simulink model "Optimate_PhysicalArchi"  (R2022b)
settings: Solver=VariableStepAuto  StartTime=0.0  StopTime=10.0  RelTol=1e-3
settings Model: DataDictionary=Optimate_PhysicalArchiDD.sldd  Creator=TO41629  LastModifiedBy=TO41629

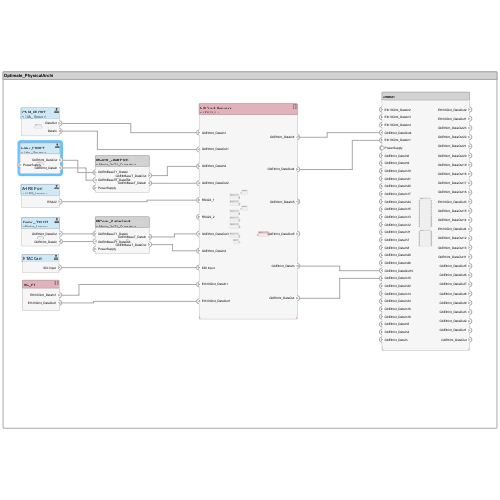
[thumbnail: Simulink's stored preview of the top-level diagram]
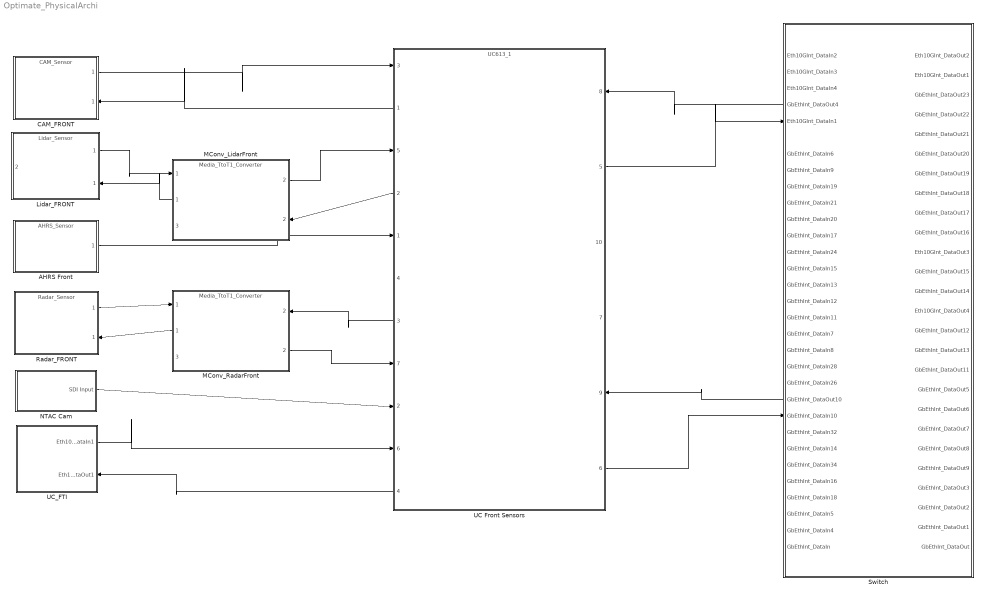
== system Optimate_PhysicalArchi ==
  AHRS Front : ModelReference  ModelNameDialog=AHRS_Sensor  SimulationMode=Normal  ModelReferenceVersion=1.2
      settings: PortSchema="{\"entries\":[{\"content\":{\"headerSize\":38,\"margin\":15,\"minimumSpacing\":25,\"sides\":[{\"content\":{\"connectorIds\":[]},\"type\":\"ConnectorPlacement.EquallySpacedRectSide\",\"uuid\":\"c7a9dcc5-4699-4aa5-9b03-01cd9c9d5d35\"},{\"content\":{\"connectorIds\":[\"Out1\"],\"side\":\"RIGHT\"},\"type\":\"ConnectorPlacement.EquallySpacedRectSide\",\"uuid\":\"7085d3c2-4a9c-4f60-a450-73088e37e883\"},{\"content\":{\"connectorIds\":[],\"side\":\"TOP\"},\"type\":\"ConnectorPlacement.EquallySpacedRectSide\",\"uuid\":\"b1aea649-404c-4f50-816f-0908c9ccfd50\"}]},\"type\":\"ConnectorPlacement.EquallySpacedConnector\",\"uuid\":\"4d292e22-38cf-4a1e-b63b-51fd039b5bd2\"}],\"packageUris\":[\"http://schema.mathworks.com/mf0/Connector/R2020b\"],\"version\":\"1.0\"}"
  CAM_FRONT : ModelReference  ModelNameDialog=CAM_Sensor  UsingDefaultArgumentValue=0,0,0,0,0  SimulationMode=Normal  ModelReferenceVersion=1.17
      settings: PortSchema="{\"entries\":[{\"content\":{\"headerSize\":38,\"margin\":15,\"minimumSpacing\":25,\"sides\":[{\"content\":{\"connectorIds\":[]},\"type\":\"ConnectorPlacement.EquallySpacedRectSide\",\"uuid\":\"c7a9dcc5-4699-4aa5-9b03-01cd9c9d5d35\"},{\"content\":{\"connectorIds\":[\"Out1\",\"In1\"],\"side\":\"RIGHT\"},\"type\":\"ConnectorPlacement.EquallySpacedRectSide\",\"uuid\":\"7085d3c2-4a9c-4f60-a450-73088e37e883\"},{\"content\":{\"connectorIds\":[],\"side\":\"TOP\"},\"type\":\"ConnectorPlacement.EquallySpacedRectSide\",\"uuid\":\"b1aea649-404c-4f50-816f-0908c9ccfd50\"}]},\"type\":\"ConnectorPlacement.EquallySpacedConnector\",\"uuid\":\"4d292e22-38cf-4a1e-b63b-51fd039b5bd2\"}],\"packageUris\":[\"http://schema.mathworks.com/mf0/Connector/R2020b\"],\"version\":\"1.0\"}"
  Lidar_FRONT : ModelReference  ModelNameDialog=Lidar_Sensor  SimulationMode=Normal  ModelReferenceVersion=1.6
      settings: PortSchema="{\"entries\":[{\"content\":{\"headerSize\":38,\"margin\":15,\"minimumSpacing\":25,\"sides\":[{\"content\":{\"connectorIds\":[\"In2\"]},\"type\":\"ConnectorPlacement.EquallySpacedRectSide\",\"uuid\":\"c7a9dcc5-4699-4aa5-9b03-01cd9c9d5d35\"},{\"content\":{\"connectorIds\":[\"Out1\",\"In1\"],\"side\":\"RIGHT\"},\"type\":\"ConnectorPlacement.EquallySpacedRectSide\",\"uuid\":\"7085d3c2-4a9c-4f60-a450-73088e37e883\"},{\"content\":{\"connectorIds\":[],\"side\":\"TOP\"},\"type\":\"ConnectorPlacement.EquallySpacedRectSide\",\"uuid\":\"b1aea649-404c-4f50-816f-0908c9ccfd50\"}]},\"type\":\"ConnectorPlacement.EquallySpacedConnector\",\"uuid\":\"4d292e22-38cf-4a1e-b63b-51fd039b5bd2\"}],\"packageUris\":[\"http://schema.mathworks.com/mf0/Connector/R2020b\"],\"version\":\"1.0\"}"
  MConv_LidarFront : ModelReference  ModelNameDialog=Media_TtoT1_Converter  SimulationMode=Normal  ModelReferenceVersion=1.4
      settings: PortSchema="{\"entries\":[{\"content\":{\"headerSize\":38,\"margin\":15,\"minimumSpacing\":25,\"sides\":[{\"content\":{\"connectorIds\":[\"In1\",\"Out1\",\"In3\"]},\"type\":\"ConnectorPlacement.EquallySpacedRectSide\",\"uuid\":\"99f9264f-b53d-4971-8b33-a510fd21d3a3\"},{\"content\":{\"connectorIds\":[\"Out2\",\"In2\"],\"side\":\"RIGHT\"},\"type\":\"ConnectorPlacement.EquallySpacedRectSide\",\"uuid\":\"2d9ba29c-7f97-48cb-9608-186fea073d48\"},{\"content\":{\"connectorIds\":[],\"side\":\"TOP\"},\"type\":\"ConnectorPlacement.EquallySpacedRectSide\",\"uuid\":\"4aabfdd9-8cc9-4862-a428-8fddf83f7eb0\"}]},\"type\":\"ConnectorPlacement.EquallySpacedConnector\",\"uuid\":\"0c6b3b40-bc47-4abe-952f-60d13c7625c4\"}],\"packageUris\":[\"http://schema.mathworks.com/mf0/Connector/R2020b\"],\"version\":\"1.0\"}"
  MConv_RadarFront : ModelReference  ModelNameDialog=Media_TtoT1_Converter  SimulationMode=Normal  ModelReferenceVersion=1.4
      settings: PortSchema="{\"entries\":[{\"content\":{\"headerSize\":38,\"margin\":15,\"minimumSpacing\":25,\"sides\":[{\"content\":{\"connectorIds\":[\"In1\",\"Out1\",\"In3\"]},\"type\":\"ConnectorPlacement.EquallySpacedRectSide\",\"uuid\":\"99f9264f-b53d-4971-8b33-a510fd21d3a3\"},{\"content\":{\"connectorIds\":[\"In2\",\"Out2\"],\"side\":\"RIGHT\"},\"type\":\"ConnectorPlacement.EquallySpacedRectSide\",\"uuid\":\"2d9ba29c-7f97-48cb-9608-186fea073d48\"},{\"content\":{\"connectorIds\":[],\"side\":\"TOP\"},\"type\":\"ConnectorPlacement.EquallySpacedRectSide\",\"uuid\":\"4aabfdd9-8cc9-4862-a428-8fddf83f7eb0\"}]},\"type\":\"ConnectorPlacement.EquallySpacedConnector\",\"uuid\":\"0c6b3b40-bc47-4abe-952f-60d13c7625c4\"}],\"packageUris\":[\"http://schema.mathworks.com/mf0/Connector/R2020b\"],\"version\":\"1.0\"}"
  NTAC Cam : Subsystem
      settings: PortSchema="{\"entries\":[{\"content\":{\"headerSize\":26,\"margin\":15,\"minimumSpacing\":25,\"sides\":[{\"content\":{\"connectorIds\":[]},\"type\":\"ConnectorPlacement.EquallySpacedRectSide\",\"uuid\":\"c7a9dcc5-4699-4aa5-9b03-01cd9c9d5d35\"},{\"content\":{\"connectorIds\":[\"Out1\"],\"side\":\"RIGHT\"},\"type\":\"ConnectorPlacement.EquallySpacedRectSide\",\"uuid\":\"7085d3c2-4a9c-4f60-a450-73088e37e883\"},{\"content\":{\"connectorIds\":[],\"side\":\"TOP\"},\"type\":\"ConnectorPlacement.EquallySpacedRectSide\",\"uuid\":\"b1aea649-404c-4f50-816f-0908c9ccfd50\"}]},\"type\":\"ConnectorPlacement.EquallySpacedConnector\",\"uuid\":\"4d292e22-38cf-4a1e-b63b-51fd039b5bd2\"}],\"packageUris\":[\"http://schema.mathworks.com/mf0/Connector/R2020b\"],\"version\":\"1.0\"}"
  Radar_FRONT : ModelReference  ModelNameDialog=Radar_Sensor  UsingDefaultArgumentValue=0,0,0  SimulationMode=Normal  ModelReferenceVersion=1.5
      settings: PortSchema="{\"entries\":[{\"content\":{\"headerSize\":38,\"margin\":15,\"minimumSpacing\":25,\"sides\":[{\"content\":{\"connectorIds\":[]},\"type\":\"ConnectorPlacement.EquallySpacedRectSide\",\"uuid\":\"c7a9dcc5-4699-4aa5-9b03-01cd9c9d5d35\"},{\"content\":{\"connectorIds\":[\"Out1\",\"In1\"],\"side\":\"RIGHT\"},\"type\":\"ConnectorPlacement.EquallySpacedRectSide\",\"uuid\":\"7085d3c2-4a9c-4f60-a450-73088e37e883\"},{\"content\":{\"connectorIds\":[],\"side\":\"TOP\"},\"type\":\"ConnectorPlacement.EquallySpacedRectSide\",\"uuid\":\"b1aea649-404c-4f50-816f-0908c9ccfd50\"}]},\"type\":\"ConnectorPlacement.EquallySpacedConnector\",\"uuid\":\"4d292e22-38cf-4a1e-b63b-51fd039b5bd2\"}],\"packageUris\":[\"http://schema.mathworks.com/mf0/Connector/R2020b\"],\"version\":\"1.0\"}"
  Switch : Subsystem
      settings: PortSchema="{\"entries\":[{\"content\":{\"headerSize\":26,\"margin\":15,\"minimumSpacing\":25,\"sides\":[{\"content\":{\"connectorIds\":[\"In1\",\"In2\",\"In3\",\"Out24\",\"In4\",\"LConn1\",\"In5\",\"In6\",\"In7\",\"In8\",\"In9\",\"In10\",\"In11\",\"In12\",\"In13\",\"In14\",\"In15\",\"In16\",\"In17\",\"In18\",\"In19\",\"Out14\",\"In20\",\"In21\",\"In22\",\"In23\",\"In24\",\"In25\",\"In26\",\"In27\",\"In28\"]},\"type\":\"ConnectorPlacement.EquallySpacedRectSide\",\"uuid\":\"c7a9dcc5-4699-4aa5-9b03-01cd9c9d5d35\"},{\"content\":{\"connectorIds\":[\"Out1\",\"Out2\",\"Out3\",\"Out4\",\"Out5\",\"Out6\",\"Out7\",\"Out8\",\"Out9\",\"Out10\",\"Out11\",\"Out12\",\"Out13\",\"Out15\",\"Out16\",\"Out17\",\"Out18\",\"Out19\",\"Out20\",\"Out21\",\"Out22\",\"Out23\",\"Out25\",\"Out26\",\"Out27\",\"Out28\"],\"side\":\"RIGHT\"},\"type\":\"ConnectorPlacement.EquallySpacedRectSide\",\"uuid\":\"7085d3c2-4a9c-4f60-a450-73088e37e883\"},{\"content\":{\"connectorIds\":[],\"side\":\"TOP\"},\"type\":\"ConnectorPlacement.EquallySpacedRectSide\",\"uuid\":\"b1aea649-404c-4f50-816f-0908c9ccfd50\"}]},\"type\":\"ConnectorPlacement.EquallySpacedConnector\",\"uuid\":\"4d292e22-38cf-4a1e-b63b-51fd039b5bd2\"}],\"packageUris\":[\"http://schema.mathworks.com/mf0/Connector/R2020b\"],\"version\":\"1.0\"}"
  UC Front Sensors : ModelReference  ModelNameDialog=UC613_1  UsingDefaultArgumentValue=0,0,0,0,0,0,0,0,0,0,0,0,0,0,0,0,0,0,0,0,0,0  SimulationMode=Normal  ModelReferenceVersion=1.19
      settings: PortSchema="{\"entries\":[{\"content\":{\"headerSize\":38,\"margin\":15,\"minimumSpacing\":25,\"sides\":[{\"content\":{\"connectorIds\":[\"In3\",\"Out1\",\"In5\",\"Out2\",\"In1\",\"In4\",\"Out3\",\"In7\",\"In2\",\"In6\",\"Out4\"]},\"type\":\"ConnectorPlacement.EquallySpacedRectSide\",\"uuid\":\"c7a9dcc5-4699-4aa5-9b03-01cd9c9d5d35\"},{\"content\":{\"connectorIds\":[\"In8\",\"Out5\",\"In10\",\"Out7\",\"In9\",\"Out6\"],\"side\":\"RIGHT\"},\"type\":\"ConnectorPlacement.EquallySpacedRectSide\",\"uuid\":\"7085d3c2-4a9c-4f60-a450-73088e37e883\"},{\"content\":{\"connectorIds\":[],\"side\":\"TOP\"},\"type\":\"ConnectorPlacement.EquallySpacedRectSide\",\"uuid\":\"b1aea649-404c-4f50-816f-0908c9ccfd50\"}]},\"type\":\"ConnectorPlacement.EquallySpacedConnector\",\"uuid\":\"4d292e22-38cf-4a1e-b63b-51fd039b5bd2\"}],\"packageUris\":[\"http://schema.mathworks.com/mf0/Connector/R2020b\"],\"version\":\"1.0\"}"
  UC_FTI : Subsystem  Description=|
      | UC that is managed at FTI level and is in charge of following functions:
      | - FTAC streamer for OPTIMATE Purpose.
      | - EVS recorder for Design Office purpose.
      | - EVS Streamer for OPTIMATE purpose.
      settings: PortSchema="{\"entries\":[{\"content\":{\"headerSize\":26,\"margin\":15,\"minimumSpacing\":25,\"sides\":[{\"content\":{\"connectorIds\":[]},\"type\":\"ConnectorPlacement.EquallySpacedRectSide\",\"uuid\":\"c7a9dcc5-4699-4aa5-9b03-01cd9c9d5d35\"},{\"content\":{\"connectorIds\":[\"Out1\",\"In1\"],\"side\":\"RIGHT\"},\"type\":\"ConnectorPlacement.EquallySpacedRectSide\",\"uuid\":\"7085d3c2-4a9c-4f60-a450-73088e37e883\"},{\"content\":{\"connectorIds\":[],\"side\":\"TOP\"},\"type\":\"ConnectorPlacement.EquallySpacedRectSide\",\"uuid\":\"b1aea649-404c-4f50-816f-0908c9ccfd50\"}]},\"type\":\"ConnectorPlacement.EquallySpacedConnector\",\"uuid\":\"4d292e22-38cf-4a1e-b63b-51fd039b5bd2\"}],\"packageUris\":[\"http://schema.mathworks.com/mf0/Connector/R2020b\"],\"version\":\"1.0\"}"
  wires:
  CAM_FRONT/1 -> UC Front Sensors/3
  UC Front Sensors/1 -> CAM_FRONT/1
  AHRS Front/1 -> UC Front Sensors/1
  NTAC Cam/1(SDI Input) -> UC Front Sensors/2
  UC_FTI/1(Eth10GInt_DataIn1) -> UC Front Sensors/6
  UC Front Sensors/4 -> UC_FTI/1(Eth10GInt_DataOut1)
  UC Front Sensors/3 -> MConv_RadarFront/2
  MConv_RadarFront/2 -> UC Front Sensors/7
  Radar_FRONT/1 -> MConv_RadarFront/1
  MConv_RadarFront/1 -> Radar_FRONT/1
  MConv_LidarFront/2 -> UC Front Sensors/5
  UC Front Sensors/2 -> MConv_LidarFront/2
  Lidar_FRONT/1 -> MConv_LidarFront/1
  MConv_LidarFront/1 -> Lidar_FRONT/1
  UC Front Sensors/5 -> Switch/4(Eth10GInt_DataIn1)
  Switch/24(GbEthInt_DataOut4) -> UC Front Sensors/8
  UC Front Sensors/6 -> Switch/20(GbEthInt_DataIn10)
  Switch/14(GbEthInt_DataOut10) -> UC Front Sensors/9

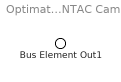
== system Optimate_PhysicalArchi/NTAC Cam ==
  Bus Element Out1 : Outport  PortName=SDI Input

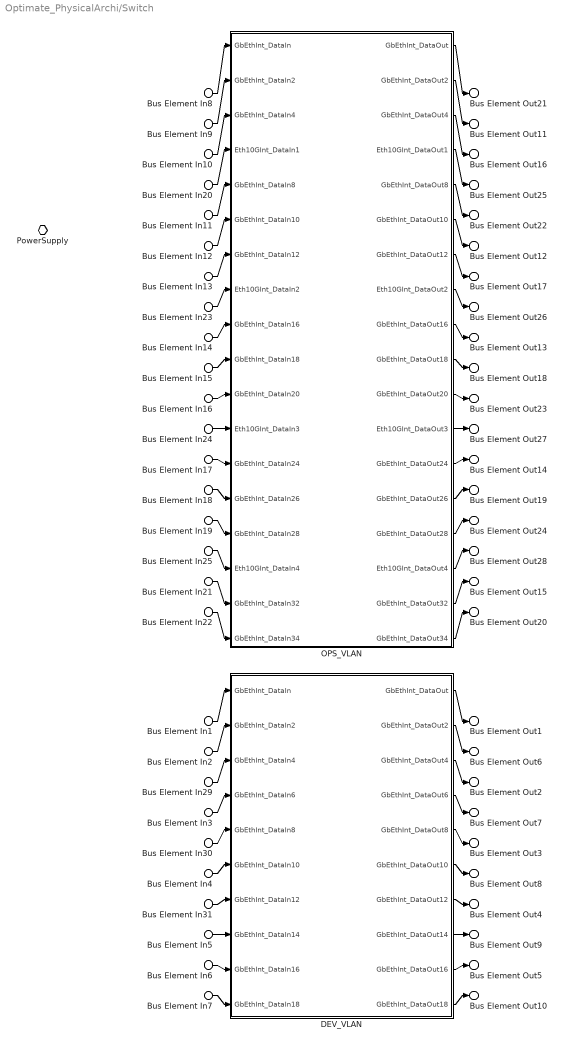
== system Optimate_PhysicalArchi/Switch ==
  Bus Element In23 : Inport  PortName=Eth10GInt_DataIn2
  Bus Element In24 : Inport  Port=2  PortName=Eth10GInt_DataIn3
  Bus Element In25 : Inport  Port=3  PortName=Eth10GInt_DataIn4
  Bus Element In20 : Inport  Port=4  PortName=Eth10GInt_DataIn1
  Bus Element In31 : Inport  Port=5  PortName=GbEthInt_DataIn6
  Bus Element In8 : Inport  Port=6  PortName=GbEthInt_DataIn9
  Bus Element In14 : Inport  Port=7  PortName=GbEthInt_DataIn19
  Bus Element In16 : Inport  Port=8  PortName=GbEthInt_DataIn21
  Bus Element In15 : Inport  Port=9  PortName=GbEthInt_DataIn20
  Bus Element In13 : Inport  Port=10  PortName=GbEthInt_DataIn17
  Bus Element In17 : Inport  Port=11  PortName=GbEthInt_DataIn24
  Bus Element In12 : Inport  Port=12  PortName=GbEthInt_DataIn15
  Bus Element In11 : Inport  Port=13  PortName=GbEthInt_DataIn13
  Bus Element In10 : Inport  Port=14  PortName=GbEthInt_DataIn12
  Bus Element In9 : Inport  Port=15  PortName=GbEthInt_DataIn11
  Bus Element In2 : Inport  Port=16  PortName=GbEthInt_DataIn7
  Bus Element In3 : Inport  Port=17  PortName=GbEthInt_DataIn8
  Bus Element In19 : Inport  Port=18  PortName=GbEthInt_DataIn28
  Bus Element In18 : Inport  Port=19  PortName=GbEthInt_DataIn26
  Bus Element In4 : Inport  Port=20  PortName=GbEthInt_DataIn10
  Bus Element In21 : Inport  Port=21  PortName=GbEthInt_DataIn32
  Bus Element In5 : Inport  Port=22  PortName=GbEthInt_DataIn14
  Bus Element In22 : Inport  Port=23  PortName=GbEthInt_DataIn34
  Bus Element In6 : Inport  Port=24  PortName=GbEthInt_DataIn16
  Bus Element In7 : Inport  Port=25  PortName=GbEthInt_DataIn18
  Bus Element In30 : Inport  Port=26  PortName=GbEthInt_DataIn5
  Bus Element In29 : Inport  Port=27  PortName=GbEthInt_DataIn4
  Bus Element In1 : Inport  Port=28  PortName=GbEthInt_DataIn
  DEV_VLAN : Subsystem
      settings: PortSchema="{\"entries\":[{\"content\":{\"headerSize\":26,\"margin\":15,\"minimumSpacing\":25,\"sides\":[{\"content\":{\"connectorIds\":[\"In1\",\"In2\",\"In3\",\"In4\",\"In5\",\"In6\",\"In7\",\"In8\",\"In9\",\"In10\"]},\"type\":\"ConnectorPlacement.EquallySpacedRectSide\",\"uuid\":\"e7200d3e-a7a3-4553-990a-a5a081142ec7\"},{\"content\":{\"connectorIds\":[\"Out1\",\"Out2\",\"Out3\",\"Out4\",\"Out5\",\"Out6\",\"Out7\",\"Out8\",\"Out9\",\"Out10\"],\"side\":\"RIGHT\"},\"type\":\"ConnectorPlacement.EquallySpacedRectSide\",\"uuid\":\"8929064b-436b-4590-8edd-485d8e65b6e0\"},{\"content\":{\"connectorIds\":[],\"side\":\"TOP\"},\"type\":\"ConnectorPlacement.EquallySpacedRectSide\",\"uuid\":\"bbdc2cfb-ca63-45b7-bc30-3813769456c1\"}]},\"type\":\"ConnectorPlacement.EquallySpacedConnector\",\"uuid\":\"d9e8dfb7-77d1-4fb7-804b-637895c6daf0\"}],\"packageUris\":[\"http://schema.mathworks.com/mf0/Connector/R2020b\"],\"version\":\"1.0\"}"
  OPS_VLAN : Subsystem
      settings: PortSchema="{\"entries\":[{\"content\":{\"headerSize\":26,\"margin\":15,\"minimumSpacing\":25,\"sides\":[{\"content\":{\"connectorIds\":[\"In1\",\"In2\",\"In3\",\"In4\",\"In5\",\"In6\",\"In7\",\"In8\",\"In9\",\"In10\",\"In11\",\"In12\",\"In13\",\"In14\",\"In15\",\"In16\",\"In17\",\"In18\"]},\"type\":\"ConnectorPlacement.EquallySpacedRectSide\",\"uuid\":\"e7200d3e-a7a3-4553-990a-a5a081142ec7\"},{\"content\":{\"connectorIds\":[\"Out1\",\"Out2\",\"Out3\",\"Out4\",\"Out5\",\"Out6\",\"Out7\",\"Out8\",\"Out9\",\"Out10\",\"Out11\",\"Out12\",\"Out13\",\"Out14\",\"Out15\",\"Out16\",\"Out17\",\"Out18\"],\"side\":\"RIGHT\"},\"type\":\"ConnectorPlacement.EquallySpacedRectSide\",\"uuid\":\"8929064b-436b-4590-8edd-485d8e65b6e0\"},{\"content\":{\"connectorIds\":[],\"side\":\"TOP\"},\"type\":\"ConnectorPlacement.EquallySpacedRectSide\",\"uuid\":\"bbdc2cfb-ca63-45b7-bc30-3813769456c1\"}]},\"type\":\"ConnectorPlacement.EquallySpacedConnector\",\"uuid\":\"d9e8dfb7-77d1-4fb7-804b-637895c6daf0\"}],\"packageUris\":[\"http://schema.mathworks.com/mf0/Connector/R2020b\"],\"version\":\"1.0\"}"
  PowerSupply : PMIOPort  Side=Left
  Bus Element Out26 : Outport  PortName=Eth10GInt_DataOut2
  Bus Element Out25 : Outport  Port=2  PortName=Eth10GInt_DataOut1
  Bus Element Out24 : Outport  Port=3  PortName=GbEthInt_DataOut23
  Bus Element Out23 : Outport  Port=4  PortName=GbEthInt_DataOut22
  Bus Element Out22 : Outport  Port=5  PortName=GbEthInt_DataOut21
  Bus Element Out21 : Outport  Port=6  PortName=GbEthInt_DataOut20
  Bus Element Out20 : Outport  Port=7  PortName=GbEthInt_DataOut19
  Bus Element Out19 : Outport  Port=8  PortName=GbEthInt_DataOut18
  Bus Element Out18 : Outport  Port=9  PortName=GbEthInt_DataOut17
  Bus Element Out17 : Outport  Port=10  PortName=GbEthInt_DataOut16
  Bus Element Out27 : Outport  Port=11  PortName=Eth10GInt_DataOut3
  Bus Element Out16 : Outport  Port=12  PortName=GbEthInt_DataOut15
  Bus Element Out15 : Outport  Port=13  PortName=GbEthInt_DataOut14
  Bus Element Out11 : Outport  Port=14  PortName=GbEthInt_DataOut10
  Bus Element Out28 : Outport  Port=15  PortName=Eth10GInt_DataOut4
  Bus Element Out13 : Outport  Port=16  PortName=GbEthInt_DataOut12
  Bus Element Out14 : Outport  Port=17  PortName=GbEthInt_DataOut13
  Bus Element Out12 : Outport  Port=18  PortName=GbEthInt_DataOut11
  Bus Element Out6 : Outport  Port=19  PortName=GbEthInt_DataOut5
  Bus Element Out7 : Outport  Port=20  PortName=GbEthInt_DataOut6
  Bus Element Out8 : Outport  Port=21  PortName=GbEthInt_DataOut7
  Bus Element Out9 : Outport  Port=22  PortName=GbEthInt_DataOut8
  Bus Element Out10 : Outport  Port=23  PortName=GbEthInt_DataOut9
  Bus Element Out5 : Outport  Port=24  PortName=GbEthInt_DataOut4
  Bus Element Out4 : Outport  Port=25  PortName=GbEthInt_DataOut3
  Bus Element Out3 : Outport  Port=26  PortName=GbEthInt_DataOut2
  Bus Element Out2 : Outport  Port=27  PortName=GbEthInt_DataOut1
  Bus Element Out1 : Outport  Port=28  PortName=GbEthInt_DataOut
  wires:
  OPS_VLAN/6(GbEthInt_DataOut10) -> Bus Element Out12/1
  Bus Element In9/1 -> OPS_VLAN/2(GbEthInt_DataIn2)
  Bus Element In8/1 -> OPS_VLAN/1(GbEthInt_DataIn)
  Bus Element In11/1 -> OPS_VLAN/5(GbEthInt_DataIn8)
  Bus Element In10/1 -> OPS_VLAN/3(GbEthInt_DataIn4)
  Bus Element In29/1 -> DEV_VLAN/3(GbEthInt_DataIn4)
  Bus Element In22/1 -> OPS_VLAN/18(GbEthInt_DataIn34)
  Bus Element In12/1 -> OPS_VLAN/6(GbEthInt_DataIn10)
  Bus Element In13/1 -> OPS_VLAN/7(GbEthInt_DataIn12)
  Bus Element In14/1 -> OPS_VLAN/9(GbEthInt_DataIn16)
  Bus Element In3/1 -> DEV_VLAN/4(GbEthInt_DataIn6)
  Bus Element In15/1 -> OPS_VLAN/10(GbEthInt_DataIn18)
  Bus Element In16/1 -> OPS_VLAN/11(GbEthInt_DataIn20)
  OPS_VLAN/15(GbEthInt_DataOut28) -> Bus Element Out24/1
  Bus Element In17/1 -> OPS_VLAN/13(GbEthInt_DataIn24)
  OPS_VLAN/13(GbEthInt_DataOut24) -> Bus Element Out14/1
  Bus Element In19/1 -> OPS_VLAN/15(GbEthInt_DataIn28)
  Bus Element In18/1 -> OPS_VLAN/14(GbEthInt_DataIn26)
  Bus Element In4/1 -> DEV_VLAN/6(GbEthInt_DataIn10)
  DEV_VLAN/5(GbEthInt_DataOut8) -> Bus Element Out3/1
  Bus Element In21/1 -> OPS_VLAN/17(GbEthInt_DataIn32)
  Bus Element In1/1 -> DEV_VLAN/1(GbEthInt_DataIn)
  DEV_VLAN/6(GbEthInt_DataOut10) -> Bus Element Out8/1
  Bus Element In2/1 -> DEV_VLAN/2(GbEthInt_DataIn2)
  Bus Element In30/1 -> DEV_VLAN/5(GbEthInt_DataIn8)
  DEV_VLAN/9(GbEthInt_DataOut16) -> Bus Element Out5/1
  Bus Element In31/1 -> DEV_VLAN/7(GbEthInt_DataIn12)
  Bus Element In5/1 -> DEV_VLAN/8(GbEthInt_DataIn14)
  Bus Element In6/1 -> DEV_VLAN/9(GbEthInt_DataIn16)
  Bus Element In7/1 -> DEV_VLAN/10(GbEthInt_DataIn18)
  OPS_VLAN/1(GbEthInt_DataOut) -> Bus Element Out21/1
  OPS_VLAN/2(GbEthInt_DataOut2) -> Bus Element Out11/1
  OPS_VLAN/3(GbEthInt_DataOut4) -> Bus Element Out16/1
  OPS_VLAN/5(GbEthInt_DataOut8) -> Bus Element Out22/1
  OPS_VLAN/7(GbEthInt_DataOut12) -> Bus Element Out17/1
  OPS_VLAN/9(GbEthInt_DataOut16) -> Bus Element Out13/1
  OPS_VLAN/10(GbEthInt_DataOut18) -> Bus Element Out18/1
  OPS_VLAN/11(GbEthInt_DataOut20) -> Bus Element Out23/1
  OPS_VLAN/14(GbEthInt_DataOut26) -> Bus Element Out19/1
  OPS_VLAN/17(GbEthInt_DataOut32) -> Bus Element Out15/1
  OPS_VLAN/18(GbEthInt_DataOut34) -> Bus Element Out20/1
  DEV_VLAN/1(GbEthInt_DataOut) -> Bus Element Out1/1
  DEV_VLAN/10(GbEthInt_DataOut18) -> Bus Element Out10/1
  DEV_VLAN/2(GbEthInt_DataOut2) -> Bus Element Out6/1
  DEV_VLAN/3(GbEthInt_DataOut4) -> Bus Element Out2/1
  DEV_VLAN/4(GbEthInt_DataOut6) -> Bus Element Out7/1
  DEV_VLAN/7(GbEthInt_DataOut12) -> Bus Element Out4/1
  DEV_VLAN/8(GbEthInt_DataOut14) -> Bus Element Out9/1
  OPS_VLAN/4(Eth10GInt_DataOut1) -> Bus Element Out25/1
  OPS_VLAN/8(Eth10GInt_DataOut2) -> Bus Element Out26/1
  OPS_VLAN/12(Eth10GInt_DataOut3) -> Bus Element Out27/1
  OPS_VLAN/16(Eth10GInt_DataOut4) -> Bus Element Out28/1
  Bus Element In20/1 -> OPS_VLAN/4(Eth10GInt_DataIn1)
  Bus Element In23/1 -> OPS_VLAN/8(Eth10GInt_DataIn2)
  Bus Element In24/1 -> OPS_VLAN/12(Eth10GInt_DataIn3)
  Bus Element In25/1 -> OPS_VLAN/16(Eth10GInt_DataIn4)

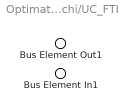
== system Optimate_PhysicalArchi/UC_FTI ==
  Bus Element In1 : Inport  PortName=Eth10GInt_DataOut1
  Bus Element Out1 : Outport  PortName=Eth10GInt_DataIn1

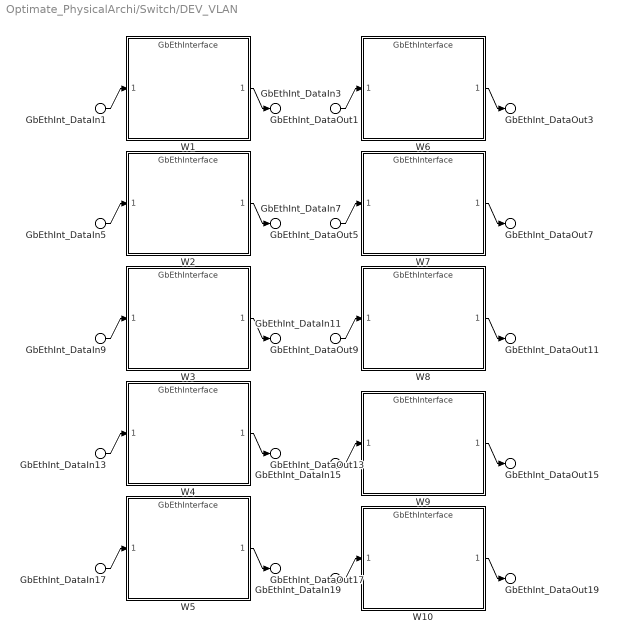
== system Optimate_PhysicalArchi/Switch/DEV_VLAN ==
  GbEthInt_DataIn1 : Inport  PortName=GbEthInt_DataIn
  GbEthInt_DataIn3 : Inport  Port=2  PortName=GbEthInt_DataIn2
  GbEthInt_DataIn5 : Inport  Port=3  PortName=GbEthInt_DataIn4
  GbEthInt_DataIn7 : Inport  Port=4  PortName=GbEthInt_DataIn6
  GbEthInt_DataIn9 : Inport  Port=5  PortName=GbEthInt_DataIn8
  GbEthInt_DataIn11 : Inport  Port=6  PortName=GbEthInt_DataIn10
  GbEthInt_DataIn13 : Inport  Port=7  PortName=GbEthInt_DataIn12
  GbEthInt_DataIn15 : Inport  Port=8  PortName=GbEthInt_DataIn14
  GbEthInt_DataIn17 : Inport  Port=9  PortName=GbEthInt_DataIn16
  GbEthInt_DataIn19 : Inport  Port=10  PortName=GbEthInt_DataIn18
  W{1..10} (10 alike) : ModelReference  ModelNameDialog=GbEthInterface  UsingDefaultArgumentValue=0,0,0  SimulationMode=Normal  ModelReferenceVersion=1.28
      settings: PortSchema="{\"entries\":[{\"content\":{\"headerSize\":38,\"margin\":15,\"minimumSpacing\":25,\"sides\":[{\"content\":{\"connectorIds\":[\"In1\"]},\"type\":\"ConnectorPlacement.EquallySpacedRectSide\",\"uuid\":\"c7a9dcc5-4699-4aa5-9b03-01cd9c9d5d35\"},{\"content\":{\"connectorIds\":[\"Out1\"],\"side\":\"RIGHT\"},\"type\":\"ConnectorPlacement.EquallySpacedRectSide\",\"uuid\":\"7085d3c2-4a9c-4f60-a450-73088e37e883\"},{\"content\":{\"connectorIds\":[],\"side\":\"TOP\"},\"type\":\"ConnectorPlacement.EquallySpacedRectSide\",\"uuid\":\"b1aea649-404c-4f50-816f-0908c9ccfd50\"}]},\"type\":\"ConnectorPlacement.EquallySpacedConnector\",\"uuid\":\"4d292e22-38cf-4a1e-b63b-51fd039b5bd2\"}],\"packageUris\":[\"http://schema.mathworks.com/mf0/Connector/R2020b\"],\"version\":\"1.0\"}"
  GbEthInt_DataOut1 : Outport  PortName=GbEthInt_DataOut
  GbEthInt_DataOut3 : Outport  Port=2  PortName=GbEthInt_DataOut2
  GbEthInt_DataOut5 : Outport  Port=3  PortName=GbEthInt_DataOut4
  GbEthInt_DataOut7 : Outport  Port=4  PortName=GbEthInt_DataOut6
  GbEthInt_DataOut9 : Outport  Port=5  PortName=GbEthInt_DataOut8
  GbEthInt_DataOut11 : Outport  Port=6  PortName=GbEthInt_DataOut10
  GbEthInt_DataOut13 : Outport  Port=7  PortName=GbEthInt_DataOut12
  GbEthInt_DataOut15 : Outport  Port=8  PortName=GbEthInt_DataOut14
  GbEthInt_DataOut17 : Outport  Port=9  PortName=GbEthInt_DataOut16
  GbEthInt_DataOut19 : Outport  Port=10  PortName=GbEthInt_DataOut18
  wires:
  W1/1 -> GbEthInt_DataOut1/1
  W6/1 -> GbEthInt_DataOut3/1
  GbEthInt_DataIn3/1 -> W6/1
  GbEthInt_DataIn9/1 -> W3/1
  W3/1 -> GbEthInt_DataOut9/1
  GbEthInt_DataIn7/1 -> W7/1
  W4/1 -> GbEthInt_DataOut13/1
  W5/1 -> GbEthInt_DataOut17/1
  GbEthInt_DataIn13/1 -> W4/1
  W10/1 -> GbEthInt_DataOut19/1
  W8/1 -> GbEthInt_DataOut11/1
  GbEthInt_DataIn1/1 -> W1/1
  W7/1 -> GbEthInt_DataOut7/1
  W2/1 -> GbEthInt_DataOut5/1
  GbEthInt_DataIn5/1 -> W2/1
  GbEthInt_DataIn17/1 -> W5/1
  GbEthInt_DataIn11/1 -> W8/1
  GbEthInt_DataIn15/1 -> W9/1
  GbEthInt_DataIn19/1 -> W10/1
  W9/1 -> GbEthInt_DataOut15/1

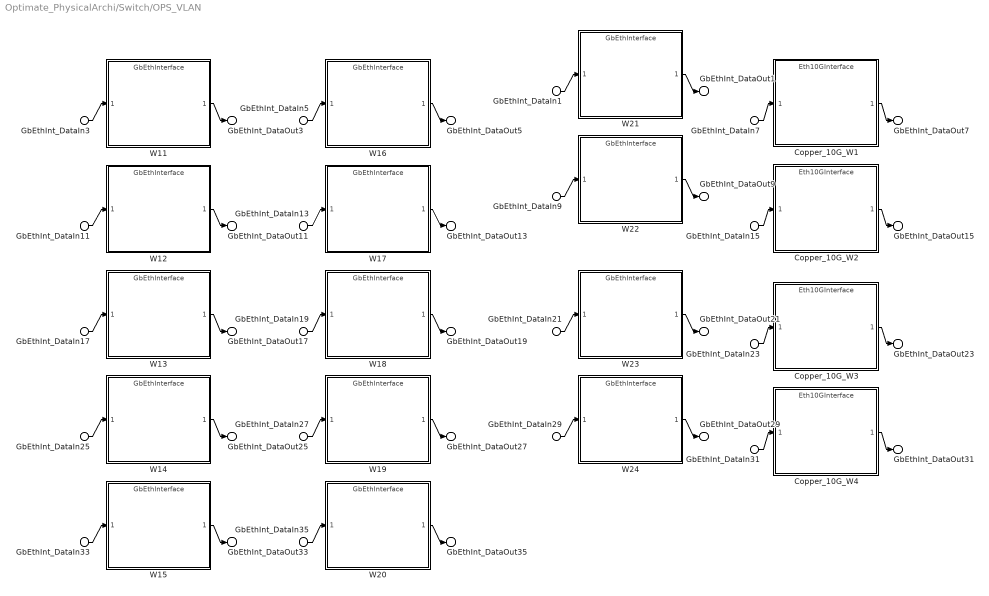
== system Optimate_PhysicalArchi/Switch/OPS_VLAN ==
  GbEthInt_DataIn1 : Inport  PortName=GbEthInt_DataIn
  GbEthInt_DataIn3 : Inport  Port=2  PortName=GbEthInt_DataIn2
  GbEthInt_DataIn5 : Inport  Port=3  PortName=GbEthInt_DataIn4
  GbEthInt_DataIn7 : Inport  Port=4  PortName=Eth10GInt_DataIn1
  GbEthInt_DataIn9 : Inport  Port=5  PortName=GbEthInt_DataIn8
  GbEthInt_DataIn11 : Inport  Port=6  PortName=GbEthInt_DataIn10
  GbEthInt_DataIn13 : Inport  Port=7  PortName=GbEthInt_DataIn12
  GbEthInt_DataIn15 : Inport  Port=8  PortName=Eth10GInt_DataIn2
  GbEthInt_DataIn17 : Inport  Port=9  PortName=GbEthInt_DataIn16
  GbEthInt_DataIn19 : Inport  Port=10  PortName=GbEthInt_DataIn18
  GbEthInt_DataIn21 : Inport  Port=11  PortName=GbEthInt_DataIn20
  GbEthInt_DataIn23 : Inport  Port=12  PortName=Eth10GInt_DataIn3
  GbEthInt_DataIn25 : Inport  Port=13  PortName=GbEthInt_DataIn24
  GbEthInt_DataIn27 : Inport  Port=14  PortName=GbEthInt_DataIn26
  GbEthInt_DataIn29 : Inport  Port=15  PortName=GbEthInt_DataIn28
  GbEthInt_DataIn31 : Inport  Port=16  PortName=Eth10GInt_DataIn4
  GbEthInt_DataIn33 : Inport  Port=17  PortName=GbEthInt_DataIn32
  GbEthInt_DataIn35 : Inport  Port=18  PortName=GbEthInt_DataIn34
  Copper_10G_W{1..4} (4 alike) : ModelReference  ModelNameDialog=Eth10GInterface  UsingDefaultArgumentValue=0,0,0  SimulationMode=Normal  ModelReferenceVersion=1.28
      settings: PortSchema="{\"entries\":[{\"content\":{\"headerSize\":38,\"margin\":15,\"minimumSpacing\":25,\"sides\":[{\"content\":{\"connectorIds\":[\"In1\"]},\"type\":\"ConnectorPlacement.EquallySpacedRectSide\",\"uuid\":\"c7a9dcc5-4699-4aa5-9b03-01cd9c9d5d35\"},{\"content\":{\"connectorIds\":[\"Out1\"],\"side\":\"RIGHT\"},\"type\":\"ConnectorPlacement.EquallySpacedRectSide\",\"uuid\":\"7085d3c2-4a9c-4f60-a450-73088e37e883\"},{\"content\":{\"connectorIds\":[],\"side\":\"TOP\"},\"type\":\"ConnectorPlacement.EquallySpacedRectSide\",\"uuid\":\"b1aea649-404c-4f50-816f-0908c9ccfd50\"}]},\"type\":\"ConnectorPlacement.EquallySpacedConnector\",\"uuid\":\"4d292e22-38cf-4a1e-b63b-51fd039b5bd2\"}],\"packageUris\":[\"http://schema.mathworks.com/mf0/Connector/R2020b\"],\"version\":\"1.0\"}"
  W{11..24} (14 alike) : ModelReference  ModelNameDialog=GbEthInterface  UsingDefaultArgumentValue=0,0,0  SimulationMode=Normal  ModelReferenceVersion=1.28
      settings: PortSchema="{\"entries\":[{\"content\":{\"headerSize\":38,\"margin\":15,\"minimumSpacing\":25,\"sides\":[{\"content\":{\"connectorIds\":[\"In1\"]},\"type\":\"ConnectorPlacement.EquallySpacedRectSide\",\"uuid\":\"c7a9dcc5-4699-4aa5-9b03-01cd9c9d5d35\"},{\"content\":{\"connectorIds\":[\"Out1\"],\"side\":\"RIGHT\"},\"type\":\"ConnectorPlacement.EquallySpacedRectSide\",\"uuid\":\"7085d3c2-4a9c-4f60-a450-73088e37e883\"},{\"content\":{\"connectorIds\":[],\"side\":\"TOP\"},\"type\":\"ConnectorPlacement.EquallySpacedRectSide\",\"uuid\":\"b1aea649-404c-4f50-816f-0908c9ccfd50\"}]},\"type\":\"ConnectorPlacement.EquallySpacedConnector\",\"uuid\":\"4d292e22-38cf-4a1e-b63b-51fd039b5bd2\"}],\"packageUris\":[\"http://schema.mathworks.com/mf0/Connector/R2020b\"],\"version\":\"1.0\"}"
  GbEthInt_DataOut1 : Outport  PortName=GbEthInt_DataOut
  GbEthInt_DataOut3 : Outport  Port=2  PortName=GbEthInt_DataOut2
  GbEthInt_DataOut5 : Outport  Port=3  PortName=GbEthInt_DataOut4
  GbEthInt_DataOut7 : Outport  Port=4  PortName=Eth10GInt_DataOut1
  GbEthInt_DataOut9 : Outport  Port=5  PortName=GbEthInt_DataOut8
  GbEthInt_DataOut11 : Outport  Port=6  PortName=GbEthInt_DataOut10
  GbEthInt_DataOut13 : Outport  Port=7  PortName=GbEthInt_DataOut12
  GbEthInt_DataOut15 : Outport  Port=8  PortName=Eth10GInt_DataOut2
  GbEthInt_DataOut17 : Outport  Port=9  PortName=GbEthInt_DataOut16
  GbEthInt_DataOut19 : Outport  Port=10  PortName=GbEthInt_DataOut18
  GbEthInt_DataOut21 : Outport  Port=11  PortName=GbEthInt_DataOut20
  GbEthInt_DataOut23 : Outport  Port=12  PortName=Eth10GInt_DataOut3
  GbEthInt_DataOut25 : Outport  Port=13  PortName=GbEthInt_DataOut24
  GbEthInt_DataOut27 : Outport  Port=14  PortName=GbEthInt_DataOut26
  GbEthInt_DataOut29 : Outport  Port=15  PortName=GbEthInt_DataOut28
  GbEthInt_DataOut31 : Outport  Port=16  PortName=Eth10GInt_DataOut4
  GbEthInt_DataOut33 : Outport  Port=17  PortName=GbEthInt_DataOut32
  GbEthInt_DataOut35 : Outport  Port=18  PortName=GbEthInt_DataOut34
  wires:
  W13/1 -> GbEthInt_DataOut17/1
  W16/1 -> GbEthInt_DataOut5/1
  GbEthInt_DataIn19/1 -> W18/1
  W21/1 -> GbEthInt_DataOut1/1
  W14/1 -> GbEthInt_DataOut25/1
  W20/1 -> GbEthInt_DataOut35/1
  GbEthInt_DataIn13/1 -> W17/1
  GbEthInt_DataIn23/1 -> Copper_10G_W3/1
  Copper_10G_W4/1 -> GbEthInt_DataOut31/1
  GbEthInt_DataIn21/1 -> W23/1
  GbEthInt_DataIn11/1 -> W12/1
  W23/1 -> GbEthInt_DataOut21/1
  GbEthInt_DataIn9/1 -> W22/1
  GbEthInt_DataIn31/1 -> Copper_10G_W4/1
  Copper_10G_W1/1 -> GbEthInt_DataOut7/1
  GbEthInt_DataIn27/1 -> W19/1
  W15/1 -> GbEthInt_DataOut33/1
  Copper_10G_W2/1 -> GbEthInt_DataOut15/1
  W19/1 -> GbEthInt_DataOut27/1
  W24/1 -> GbEthInt_DataOut29/1
  W22/1 -> GbEthInt_DataOut9/1
  GbEthInt_DataIn5/1 -> W16/1
  W11/1 -> GbEthInt_DataOut3/1
  GbEthInt_DataIn25/1 -> W14/1
  GbEthInt_DataIn15/1 -> Copper_10G_W2/1
  GbEthInt_DataIn1/1 -> W21/1
  GbEthInt_DataIn29/1 -> W24/1
  W17/1 -> GbEthInt_DataOut13/1
  W12/1 -> GbEthInt_DataOut11/1
  GbEthInt_DataIn35/1 -> W20/1
  GbEthInt_DataIn33/1 -> W15/1
  GbEthInt_DataIn7/1 -> Copper_10G_W1/1
  GbEthInt_DataIn3/1 -> W11/1
  GbEthInt_DataIn17/1 -> W13/1
  Copper_10G_W3/1 -> GbEthInt_DataOut23/1
  W18/1 -> GbEthInt_DataOut19/1
